simulink model "SCADA"  (R2025a)
settings: Solver=FixedStepAuto  StartTime=0.0  StopTime=inf  FixedStep=0.001  RelTol=1e-3
InitFcn:
  | addpath('SCADA');
  | initFcn_SCADA;
model workspace (MAT data in the model file):
  RadSysCoeff = Simulink.Parameter
  RadSysCoeff.Value = [1 2 3 4]
  RadSysCoeff.Complexity = 'real'
  RadSysCoeff.Dimensions = [1 4]
  RadSysCoeff.DataType = 'auto'
undefined symbols (not defined in the file): daq, g, HIL_act_A_cap, HIL_act_A_rod, HIL_charge_ki, HIL_charge_kp, HIL_charge_nMax, HIL_charge_nMin, HIL_ERU_kd, HIL_ERU_ki, HIL_ERU_kp, HIL_ERU_nMax, HIL_gen_kd, HIL_gen_ki, HIL_gen_kp, HIL_gen_nMax, HIL_gen_nMin, HIL_H1T_kd, HIL_H1T_ki, HIL_H1T_kp, HIL_H1T_P1fBias, HIL_H1T_P1negCutIn, HIL_H1T_P1posCutIn, HIL_H1T_P2fBias, HIL_H1T_P2negCutIn, HIL_H1T_P2posCutIn, HIL_scale_sys, HIL_WECpump_A_cap, HIL_WECpump_A_rod, HIL_WECpump_ang2lin, HIL_WECpump_negativeCtrlLimit, HIL_WECpump_positiveCtrlLimit, National_Instruments, PCIe, rho, wave_phi, wave_S_w, WEC_A_rad, WEC_B_rad, WEC_dw, WEC_F_amp, WEC_h, WEC_I, WEC_I_inf, WEC_ICs, WEC_L_cm, WEC_L_flap, WEC_m, WEC_phi_e, WEC_T, WEC_W, WEC_w
libraries: sldrtlib x26, slpidlib x4, daqlib x1, simulink x1
(part 1 of 2)
settings Model: Creator=Jeremy  LastModifiedBy=wills224
settings DataIOCC: SaveFormat=Structure  ReturnWorkspaceOutputs=off  TimeSaveName=time  SignalLoggingName=out
settings DebuggingCC: UnderspecifiedInitializationDetection=Classic  MergeDetectMultiDrivingBlocksExec=none  UnconnectedInputMsg=warning  UnconnectedOutputMsg=warning  UnconnectedLineMsg=warning
settings ModelReferenceCC: EnableRefExpFcnMdlSchedulingChecks=on  PropagateSignalLabelsOutOfModel=off
settings RTWCC: GPUComputeCapability=3.5  DLArmComputeVersion=19.05

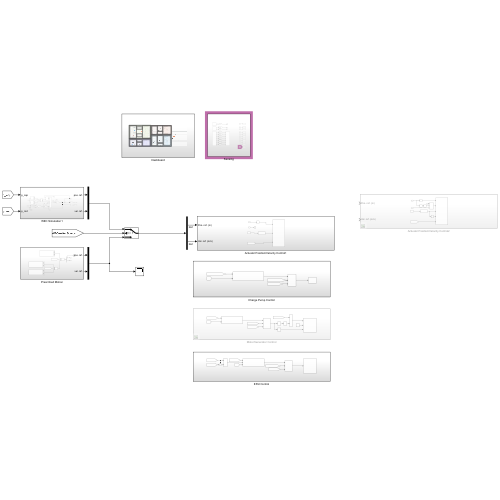
[thumbnail: Simulink's stored preview of the top-level diagram]
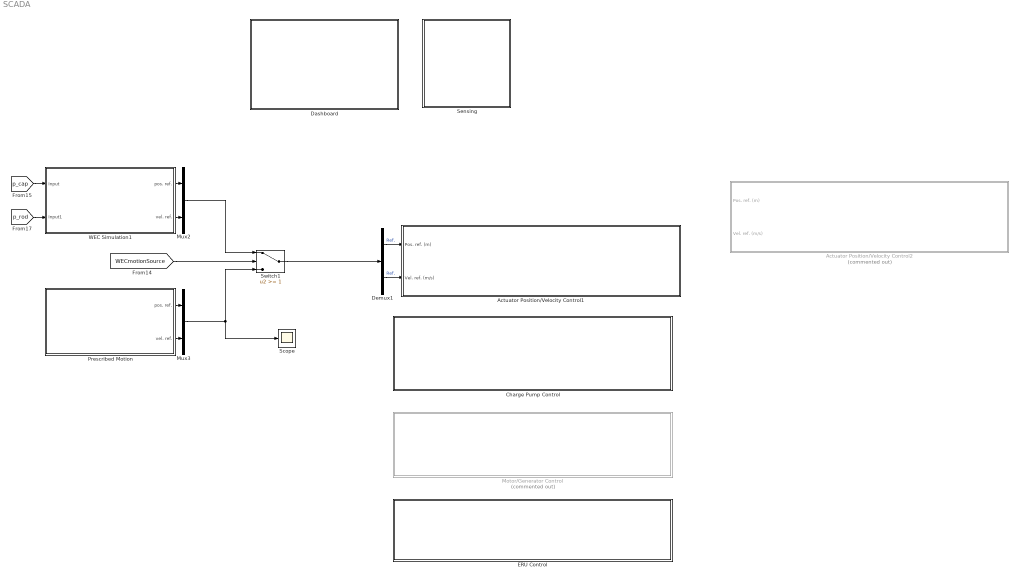
== system SCADA ==
  Actuator Position/Velocity Control1 : Subsystem
  Actuator Position/Velocity Control2 : Subsystem  Commented=on
  Charge Pump Control : Subsystem
  Dashboard : Subsystem
  Demux1 : Demux  Outputs=2
  ERU Control : Subsystem
  Motor/Generator Control : Subsystem  Commented=on
  Mux2 : Mux  Inputs=2
  Mux3 : Mux  Inputs=2
  Prescribed Motion : Subsystem
  Scope : Scope
      settings: ActiveDisplayYMinimum=-0.0625  ActiveDisplayYMaximum=0.0625  DataLoggingVariableName=ScopeData12
  Sensing : Subsystem
  Switch1 : Switch  Threshold=1  SaturateOnIntegerOverflow=off  InputSameDT=off
  WEC Simulation1 : Subsystem
  wires:
  WEC Simulation1/2(vel. ref.) -> Mux2/2
  [p_cap] -> WEC Simulation1/1(Input)
  Prescribed Motion/2(vel. ref.) -> Mux3/2
  Switch1/1 -> Demux1/1
  Demux1/2 -> Actuator Position/Velocity Control1/2(Vel. ref. (m/s))  "Ref."
  Prescribed Motion/1(pos. ref.) -> Mux3/1
  Mux3/1 -> Scope/1, Switch1/3
  [p_rod] -> WEC Simulation1/2(Input1)
  [WECmotionSource] -> Switch1/2
  WEC Simulation1/1(pos. ref.) -> Mux2/1
  Mux2/1 -> Switch1/1
  Demux1/1 -> Actuator Position/Velocity Control1/1(Pos. ref. (m))  "Ref."

== system SCADA/Actuator Position//Velocity Control1 ==
  Pos. ref. (m) : Inport
  Vel. ref. (m/s) : Inport  Port=2
  Saturation : Saturate  UpperLimit=HIL_WECpump_positiveCtrlLimit  LowerLimit=HIL_WECpump_negativeCtrlLimit
  Subsystem : Subsystem
  Terminator : Terminator
  Transfer Fcn1 : TransferFcn  Denominator=[0.001 1]
  wires:
  [x_wp] -> Transfer Fcn1/1
  Pos. ref. (m)/1 -> Saturation/1
  [H1T_shaftSpeed] -> Subsystem/3(H1T shaft speed (rpm))
  Transfer Fcn1/1 -> Subsystem/2(Pos. meas. (m))
  Saturation/1 -> Subsystem/1(Pos. ref. (m))
  Vel. ref. (m/s)/1 -> Terminator/1

== system SCADA/Actuator Position//Velocity Control2 ==
  Pos. ref. (m) : Inport
  Vel. ref. (m/s) : Inport  Port=2
  Abs : Abs  SaturateOnIntegerOverflow=off
  Constant : Constant  Value=0
  Dead Zone : DeadZone  LowerValue=HIL_WECpump_negativeCtrlLimit  UpperValue=HIL_WECpump_positiveCtrlLimit
  Derivative : Derivative
  Saturation : Saturate  UpperLimit=HIL_WECpump_positiveCtrlLimit  LowerLimit=HIL_WECpump_negativeCtrlLimit
  Subsystem : Subsystem
  Switch1 : Switch  Criteria=u2 > Threshold  SaturateOnIntegerOverflow=off  InputSameDT=off
  Transfer Fcn1 : TransferFcn  Denominator=[0.001 1]
  wires:
  Vel. ref. (m/s)/1 -> Switch1/3
  Switch1/1 -> Subsystem/2(Vel. ref. (m/s))
  Constant/1 -> Switch1/1
  Abs/1 -> Switch1/2
  Dead Zone/1 -> Abs/1
  Saturation/1 -> Subsystem/1(Pos. ref. (m))
  Transfer Fcn1/1 -> Derivative/1, Subsystem/3(Pos. meas. (m))
  [H1T_shaftSpeed] -> Subsystem/5(H1T shaft speed (rpm))
  Derivative/1 -> Subsystem/4(Vel. meas. (m/s))
  Pos. ref. (m)/1 -> Dead Zone/1, Saturation/1
  [x_wp] -> Transfer Fcn1/1

== system SCADA/Charge Pump Control ==
  Low-pressure manifold pressure control : Subsystem
  Switch : Switch  Criteria=u2 > Threshold  SaturateOnIntegerOverflow=off  InputSameDT=off
  charge pump : Subsystem
  wires:
  [p_l] -> Low-pressure manifold pressure control/2(pressure meas. (Pa))
  [ChargePumpSpeed] -> Switch/3
  [LPManifoldPressureRef] -> Low-pressure manifold pressure control/1(pressure ref. (Pa))
  Low-pressure manifold pressure control/1(charge pump shaft speed (rpm)) -> Switch/1
  [ChargePumpSpeedOrPressure] -> Switch/2
  Switch/1 -> charge pump/1(Speed ref.)

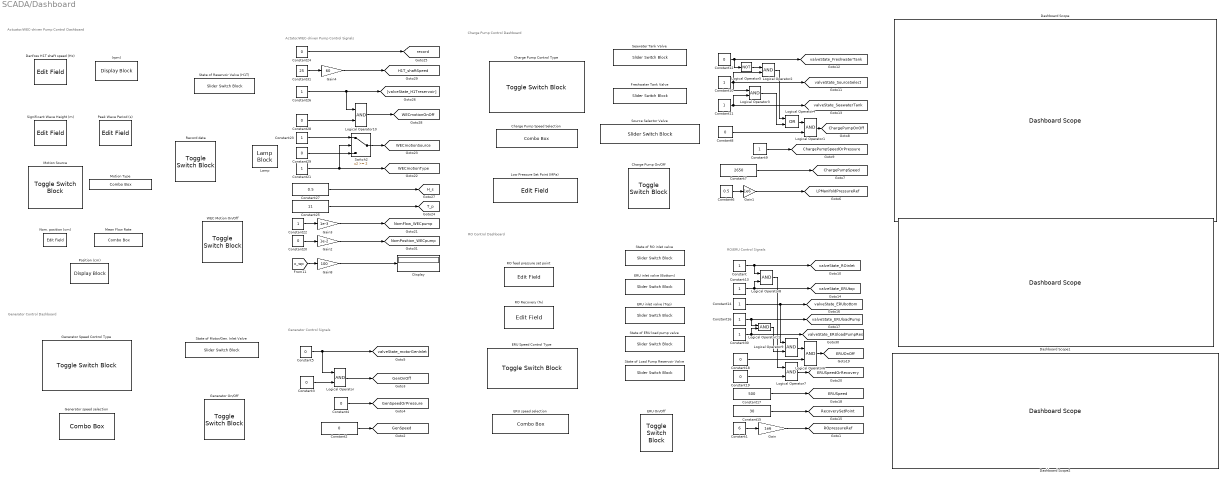
== system SCADA/Dashboard ==
  note: Charge Pump Control Dashboard
  note: Generator Control Signals
  note: RO Control Dashboard
  note: Generator Control Dashboard
  note: RO/ERU Control Signals
  note: Actator/WEC-driven Pump Control Signals
  note: Actuator/WEC-driven Pump Control Dashboard
  (rpm) : DisplayBlock  LabelPosition=Hide  Format=long  Transparency=1  GridColor=[0.502, 0.502, 0.502]
  Charge Pump Control Type : ToggleSwitchBlock  LabelPosition=Hide
  Charge Pump On/Off : ToggleSwitchBlock  LabelPosition=Hide
  Charge Pump Speed Selection : ComboBox  LabelPosition=Hide  SelectedLabel=2650 rpm
  Constant{,9..11,13..14,16,21..23,26,30} (12 alike) : Constant
  Constant1 : Constant  Value=6
  Constant{2..5,8,12,18..20,24,28..29} (12 alike) : Constant  Value=0
  Constant15 : Constant  Value=30
  Constant17 : Constant  Value=500
  Constant25 : Constant  Value=11
  Constant27 : Constant  Value=0.5
  Constant31 : Constant  Value=25
  Constant6 : Constant  Value=0.5
  Constant7 : Constant  Value=2650
  Danfoss H1T shaft speed (Hz) : EditField  LabelPosition=Hide  ShowInitialText=on  Alignment=Center
  Dashboard Scope : DashboardScope  ShowInitialText=off  FontColor=[0.0, 0.0, 0.0]
  Dashboard Scope1 : DashboardScope  FontColor=[0.0, 0.0, 0.0]
  Dashboard Scope2 : DashboardScope  FontColor=[0.0, 0.0, 0.0]
  Display : Display
  ERU On/Off : ToggleSwitchBlock  LabelPosition=Hide
  ERU Speed Control Type : ToggleSwitchBlock  LabelPosition=Hide
  ERU inlet valve (Bottom) : SliderSwitchBlock  LabelPosition=Hide
  ERU inlet valve (Top) : SliderSwitchBlock  LabelPosition=Hide
  ERU speed selection : ComboBox  LabelPosition=Hide  SelectedLabel=500 rpm
  Freshwater Tank Valve : SliderSwitchBlock  LabelPosition=Hide
  Gain : Gain  Gain=1e6
  Gain1 : Gain  Gain=1e6
  Gain2 : Gain  Gain=1e-2
  Gain3 : Gain  Gain=1e-3
  Gain4 : Gain  Gain=60
  Gain8 : Gain  Gain=100
  Generator On/Off : ToggleSwitchBlock  LabelPosition=Hide
  Generator Speed Control Type : ToggleSwitchBlock  LabelPosition=Hide
  Generator speed selection : ComboBox  LabelPosition=Hide  SelectedLabel=0 rpm
  Lamp : LampBlock  LabelPosition=Hide  DefaultColor=[192.0, 192.0, 192.0]
  Logical Operator{,1..3,6..11} (10 alike) : Logic  AllPortsSameDT=off  OutDataTypeStr=boolean
  Logical Operator4 : Logic  Operator=OR  AllPortsSameDT=off  OutDataTypeStr=boolean
  Logical Operator5 : Logic  Operator=NOT  AllPortsSameDT=off  OutDataTypeStr=boolean
  Low Pressure Set Point (MPa) : EditField  LabelPosition=Hide  ShowInitialText=on  Alignment=Center
  Mean Flow Rate : ComboBox  LabelPosition=Hide  SelectedLabel=1 L/s
  Motion Source : ToggleSwitchBlock  LabelPosition=Hide
  Motion Type : ComboBox  LabelPosition=Hide  SelectedLabel=Position, Constant
  Nom. position (cm) : EditField  LabelPosition=Hide  ShowInitialText=on  Alignment=Center
  Peak Wave Period (s) : EditField  LabelPosition=Hide  ShowInitialText=on  Alignment=Center
  Position (cm) : DisplayBlock  LabelPosition=Hide  Format=long  Transparency=1  GridColor=[0.502, 0.502, 0.502]
  RO Recovery (%) : EditField  LabelPosition=Hide  ShowInitialText=on  Alignment=Center
  RO feed pressure set point : EditField  LabelPosition=Hide  ShowInitialText=on  Alignment=Center
  Record data : ToggleSwitchBlock  LabelPosition=Hide
  Seawater Tank Valve : SliderSwitchBlock  LabelPosition=Hide
  Significant Wave Height (m) : EditField  LabelPosition=Hide  ShowInitialText=on  Alignment=Center
  Source Selector Valve : SliderSwitchBlock  LabelPosition=Hide
  State of ERU load pump valve : SliderSwitchBlock  LabelPosition=Hide
  State of Load Pump Reservoir Valve : SliderSwitchBlock  LabelPosition=Hide
  State of Motor/Gen. Inlet Valve : SliderSwitchBlock  LabelPosition=Hide
  State of RO inlet valve : SliderSwitchBlock  LabelPosition=Hide
  State of Reservoir Valve (H1T) : SliderSwitchBlock  LabelPosition=Hide
  Switch2 : Switch  Threshold=2  SaturateOnIntegerOverflow=off  InputSameDT=off
  WEC Motion On/Off : ToggleSwitchBlock  LabelPosition=Hide
  tag scope: ChargePumpOnOff=global, ChargePumpSpeed=global, ChargePumpSpeedOrPressure=global, ERUOnOff=global, ERUSpeed=global, ERUSpeedOrRecovery=global, GenOnOff=global, GenSpeed=global, GenSpeedOrPressure=global, H1T_shaftSpeed=global, H_s=global, LPManifoldPressureRef=global, NomFlow_WECpump=global, NomPosition_WECpump=global, ROpressureRef=global, RecoverySetPoint=global, T_p=global, WECmotionOnOff=global, WECmotionSource=global, WECmotionType=global, record=global, valveState_ERUbottom=global, valveState_ERUloadPump=global, valveState_ERUloadPumpRes=global, valveState_ERUtop=global, valveState_FreshwaterTank=global, valveState_ROinlet=global, valveState_SeawaterTank=global, valveState_SourceSelect=global, valveState_motorGenInlet=global
  wires:
  Constant/1 -> Logical Operator8/1, [valveState_ROinlet]
  Constant1/1 -> Gain/1
  Constant2/1 -> [GenSpeed]
  Constant3/1 -> Logical Operator/2
  Constant4/1 -> [GenSpeedOrPressure]
  Constant5/1 -> Logical Operator/1, [valveState_motorGenInlet]
  Logical Operator/1 -> [GenOnOff]
  Logical Operator1/1 -> [ChargePumpOnOff]
  Constant9/1 -> [ChargePumpSpeedOrPressure]
  Constant10/1 -> [valveState_SourceSelect], Logical Operator2/2, Logical Operator3/1
  Gain1/1 -> [LPManifoldPressureRef]
  Constant6/1 -> Gain1/1
  Constant8/1 -> Logical Operator1/2
  Constant7/1 -> [ChargePumpSpeed]
  Constant12/1 -> Logical Operator5/1, [valveState_FreshwaterTank]
  Constant11/1 -> Logical Operator3/2, [valveState_SeawaterTank]
  Logical Operator4/1 -> Logical Operator1/1
  Logical Operator3/1 -> Logical Operator4/2
  Logical Operator2/1 -> Logical Operator4/1
  Logical Operator5/1 -> Logical Operator2/1
  Logical Operator6/1 -> [ERUOnOff]
  Constant17/1 -> [ERUSpeed]
  Constant13/1 -> Logical Operator8/2, [valveState_ERUtop]
  Constant19/1 -> Logical Operator7/2
  Constant18/1 -> Logical Operator6/2
  Constant14/1 -> [valveState_ERUbottom], Logical Operator9/1
  Constant15/1 -> [RecoverySetPoint]
  Logical Operator7/1 -> [ERUSpeedOrRecovery]
  Logical Operator8/1 -> Logical Operator7/1
  Logical Operator9/1 -> Logical Operator6/1
  Constant16/1 -> [valveState_ERUloadPump], Logical Operator11/1
  Constant30/1 -> [valveState_ERUloadPumpRes], Logical Operator11/2
  Logical Operator11/1 -> Logical Operator9/2
  Gain4/1 -> [H1T_shaftSpeed]
  Constant28/1 -> Logical Operator10/2
  Constant31/1 -> Gain4/1
  Gain3/1 -> [NomFlow_WECpump]
  Logical Operator10/1 -> [WECmotionOnOff]
  Switch2/1 -> [WECmotionSource]
  Constant27/1 -> [H_s]
  Constant24/1 -> [record]
  Constant26/1 -> Logical Operator10/1, [valveState_H1Treservoir]
  Constant22/1 -> Gain3/1
  Gain2/1 -> [NomPosition_WECpump]
  Constant23/1 -> Switch2/1
  Constant29/1 -> Switch2/3
  Constant21/1 -> Switch2/2, [WECmotionType]
  Constant20/1 -> Gain2/1
  Constant25/1 -> [T_p]
  Gain8/1 -> Display/1
  [x_wp] -> Gain8/1
  Gain/1 -> [ROpressureRef]

== system SCADA/ERU Control ==
  Divide : Product  Inputs=*/
  ERU : Subsystem
  RO control : Subsystem
  Sum : Sum  Inputs=++|
  Switch : Switch  Criteria=u2 > Threshold  SaturateOnIntegerOverflow=off  InputSameDT=off
  wires:
  [p_f] -> RO control/3(feed pressure (Pa))
  [q_perm] -> Sum/1, Divide/1
  [q_brine] -> Sum/2
  Sum/1 -> Divide/2
  [RecoverySetPoint] -> RO control/1(recovery ref.)
  Divide/1 -> RO control/2(recovery meas.)
  [ERUSpeedOrRecovery] -> Switch/2
  [ERUSpeed] -> Switch/3
  RO control/1(ERU shaft speed (rpm)) -> Switch/1
  Switch/1 -> ERU/1(Speed ref.)

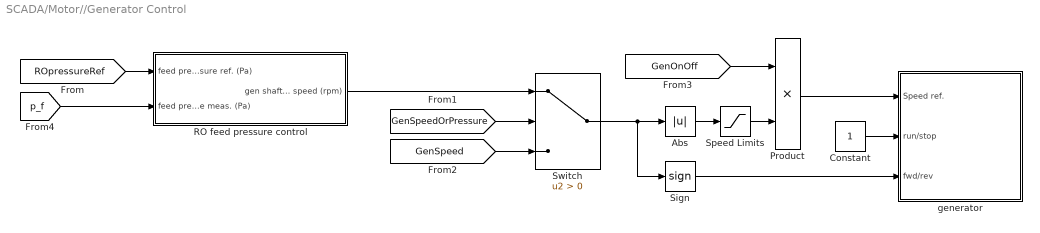
== system SCADA/Motor//Generator Control ==
  Abs : Abs  SaturateOnIntegerOverflow=off
  Constant : Constant
  Product : Product
  RO feed pressure control : Subsystem
  Sign : Signum
  Speed Limits : Saturate  UpperLimit=HIL_gen_nMax  LowerLimit=HIL_gen_nMin
  Switch : Switch  Criteria=u2 > Threshold  SaturateOnIntegerOverflow=off  InputSameDT=off
  generator : Subsystem
  wires:
  RO feed pressure control/1(gen shaft speed (rpm)) -> Switch/1
  [p_f] -> RO feed pressure control/2(feed pressure meas. (Pa))
  [ROpressureRef] -> RO feed pressure control/1(feed pressure ref. (Pa))
  Switch/1 -> Sign/1, Abs/1
  [GenSpeedOrPressure] -> Switch/2
  [GenSpeed] -> Switch/3
  [GenOnOff] -> Product/1
  Product/1 -> generator/1(Speed ref.)
  Constant/1 -> generator/2(run/stop)
  Sign/1 -> generator/3(fwd/rev)
  Speed Limits/1 -> Product/2
  Abs/1 -> Speed Limits/1

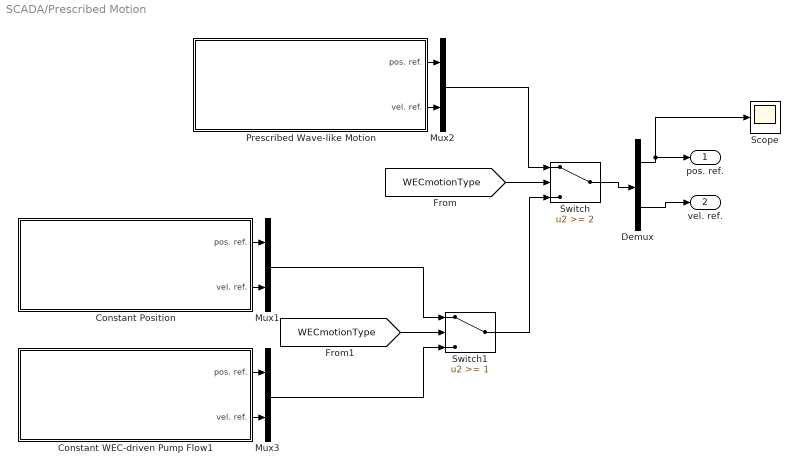
== system SCADA/Prescribed Motion ==
  Constant Position : Subsystem
  Constant WEC-driven Pump Flow1 : Subsystem
  Demux : Demux  Outputs=2
  Mux1 : Mux  Inputs=2
  Mux2 : Mux  Inputs=2
  Mux3 : Mux  Inputs=2
  Prescribed Wave-like Motion : Subsystem
  Scope : Scope
      settings: ActiveDisplayYMinimum=-0.0012499999999999976  ActiveDisplayYMaximum=0.11125  DataLoggingVariableName=ScopeData13
  Switch : Switch  Threshold=2  SaturateOnIntegerOverflow=off  InputSameDT=off
  Switch1 : Switch  Threshold=1  SaturateOnIntegerOverflow=off  InputSameDT=off
  pos. ref. : Outport
  vel. ref. : Outport  Port=2
  wires:
  Prescribed Wave-like Motion/2(vel. ref.) -> Mux2/2
  Prescribed Wave-like Motion/1(pos. ref.) -> Mux2/1
  Mux2/1 -> Switch/1
  Demux/2 -> vel. ref./1
  Demux/1 -> Scope/1, pos. ref./1
  Constant Position/1(pos. ref.) -> Mux1/1
  Constant Position/2(vel. ref.) -> Mux1/2
  [WECmotionType] -> Switch/2
  Switch/1 -> Demux/1
  Constant WEC-driven Pump Flow1/2(vel. ref.) -> Mux3/2
  Constant WEC-driven Pump Flow1/1(pos. ref.) -> Mux3/1
  Mux3/1 -> Switch1/3
  [WECmotionType] -> Switch1/2
  Switch1/1 -> Switch/3
  Mux1/1 -> Switch1/1

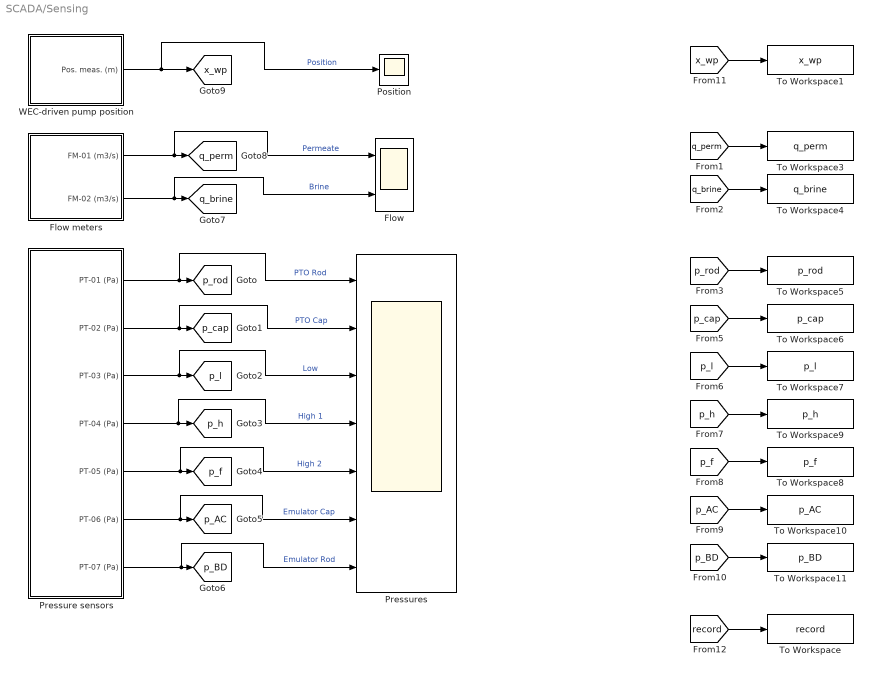
== system SCADA/Sensing ==
  Flow : Scope  NumInputPorts=2
      settings: DataLoggingVariableName=ScopeData14
  Flow meters : Subsystem
  Position : Scope
      settings: ActiveDisplayYMinimum=0.0011982402807289294  ActiveDisplayYMaximum=0.0033569285576201258  DataLoggingVariableName=ScopeData22
  Pressure sensors : Subsystem
  Pressures : Scope  NumInputPorts=7
      settings: ActiveDisplayYMinimum=-1.1076278561771905E+7  ActiveDisplayYMaximum=795336.49775385088
  To Workspace : ToWorkspace  VariableName=record  SaveFormat=Timeseries  SampleTime=-1
  To Workspace1 : ToWorkspace  VariableName=x_wp  SaveFormat=Timeseries  SampleTime=-1
  To Workspace10 : ToWorkspace  VariableName=p_AC  SaveFormat=Timeseries  SampleTime=-1
  To Workspace11 : ToWorkspace  VariableName=p_BD  SaveFormat=Timeseries  SampleTime=-1
  To Workspace3 : ToWorkspace  VariableName=q_perm  SaveFormat=Timeseries  SampleTime=-1
  To Workspace4 : ToWorkspace  VariableName=q_brine  SaveFormat=Timeseries  SampleTime=-1
  To Workspace5 : ToWorkspace  VariableName=p_rod  SaveFormat=Timeseries  SampleTime=-1
  To Workspace6 : ToWorkspace  VariableName=p_cap  SaveFormat=Timeseries  SampleTime=-1
  To Workspace7 : ToWorkspace  VariableName=p_l  SaveFormat=Timeseries  SampleTime=-1
  To Workspace8 : ToWorkspace  VariableName=p_f  SaveFormat=Timeseries  SampleTime=-1
  To Workspace9 : ToWorkspace  VariableName=p_h  SaveFormat=Timeseries  SampleTime=-1
  WEC-driven pump position : Subsystem
  tag scope: p_AC=global, p_BD=global, p_cap=global, p_f=global, p_h=global, p_l=global, p_rod=global, q_brine=global, q_perm=global, x_wp=global
  wires:
  [p_l] -> To Workspace7/1
  [p_cap] -> To Workspace6/1
  [p_h] -> To Workspace9/1
  [q_perm] -> To Workspace3/1
  [p_AC] -> To Workspace10/1
  [p_BD] -> To Workspace11/1
  [p_f] -> To Workspace8/1
  Pressure sensors/1(PT-01 (Pa)) -> Pressures/1, [p_rod]  "PTO Rod"
  Pressure sensors/4(PT-04 (Pa)) -> Pressures/4, [p_h]  "High 1"
  [q_brine] -> To Workspace4/1
  [p_rod] -> To Workspace5/1
  [x_wp] -> To Workspace1/1
  Pressure sensors/2(PT-02 (Pa)) -> Pressures/2, [p_cap]  "PTO Cap"
  [record] -> To Workspace/1
  Flow meters/2(FM-02 (m3/s)) -> Flow/2, [q_brine]  "Brine"
  Pressure sensors/3(PT-03 (Pa)) -> [p_l], Pressures/3  "Low"
  Pressure sensors/6(PT-06 (Pa)) -> Pressures/6, [p_AC]  "Emulator Cap"
  Pressure sensors/7(PT-07 (Pa)) -> Pressures/7, [p_BD]  "Emulator Rod"
  WEC-driven pump position/1(Pos. meas. (m)) -> Position/1, [x_wp]  "Position"
  Flow meters/1(FM-01 (m3/s)) -> Flow/1, [q_perm]  "Permeate"
  Pressure sensors/5(PT-05 (Pa)) -> Pressures/5, [p_f]  "High 2"

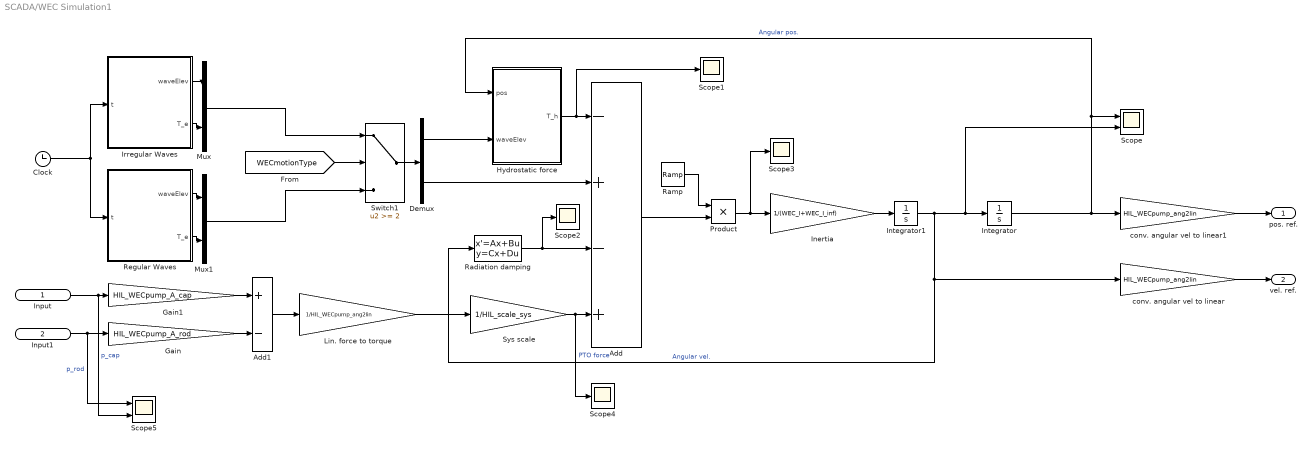
== system SCADA/WEC Simulation1 ==
  Input : Inport  SampleTime=0.01
  Input1 : Inport  Port=2  SampleTime=0.01
  Add : Sum  Inputs=-+-+
  Add1 : Sum  Inputs=+-
  Clock : Clock
  Demux : Demux  Outputs=2
  Gain : Gain  Gain=HIL_WECpump_A_rod
  Gain1 : Gain  Gain=HIL_WECpump_A_cap
  Hydrostatic force : MATLAB Function  TreatAsAtomicUnit=on
  Inertia : Gain  Gain=1/(WEC_I+WEC_I_inf)
  Integrator : Integrator
  Integrator1 : Integrator
  Irregular Waves : MATLAB Function  TreatAsAtomicUnit=on
  Lin. force to torque : Gain  Gain=1/HIL_WECpump_ang2lin
  Mux : Mux  Inputs=2
  Mux1 : Mux  Inputs=2
  Product : Product
  Radiation damping : StateSpace  A=WEC_A_rad  B=WEC_B_rad  C=[1,0,0]  D=0  InitialCondition=WEC_ICs
  Ramp : simulink/Sources/Ramp  slope=1/5  start=0.5  InitialOutput=0
  Regular Waves : MATLAB Function  TreatAsAtomicUnit=on
  Scope : Scope  NumInputPorts=2
      settings: DataLoggingSaveFormat=Array
  Scope{1..4} (4 alike) : Scope
      Scope1 settings: DataLoggingVariableName=ScopeData2  DataLoggingSaveFormat=Array
      Scope2 settings: DataLoggingVariableName=ScopeData3  DataLoggingSaveFormat=Array
      Scope3 settings: DataLoggingVariableName=ScopeData4  DataLoggingSaveFormat=Array
      Scope4 settings: DataLoggingVariableName=ScopeData5  DataLoggingSaveFormat=Array
  Scope5 : Scope  NumInputPorts=2
      settings: DataLoggingVariableName=ScopeData6  DataLoggingSaveFormat=Array
  Switch1 : Switch  Threshold=2  SaturateOnIntegerOverflow=off  InputSameDT=off
  Sys scale : Gain  Gain=1/HIL_scale_sys
  conv. angular vel to linear : Gain  Gain=HIL_WECpump_ang2lin
  conv. angular vel to linear1 : Gain  Gain=HIL_WECpump_ang2lin
  pos. ref. : Outport
  vel. ref. : Outport  Port=2
  wires:
  Radiation damping/1 -> Add/3, Scope2/1
  Clock/1 -> Regular Waves/1(t), Irregular Waves/1(t)
  Irregular Waves/1(waveElev) -> Mux/1
  Irregular Waves/2(T_e) -> Mux/2
  Hydrostatic force/1(T_h) -> Scope1/1, Add/1
  Inertia/1 -> Integrator1/1
  Integrator1/1 -> Scope/2, Integrator/1, Radiation damping/1, conv. angular vel to linear/1  "Angular vel."
  Integrator/1 -> conv. angular vel to linear1/1, Scope/1, Hydrostatic force/1(pos)  "Angular pos."
  Lin. force to torque/1 -> Sys scale/1
  Add1/1 -> Lin. force to torque/1
  Input/1 -> Scope5/2, Gain1/1  "p_cap"
  Input1/1 -> Scope5/1, Gain/1  "p_rod"
  conv. angular vel to linear1/1 -> pos. ref./1
  conv. angular vel to linear/1 -> vel. ref./1
  Sys scale/1 -> Add/4, Scope4/1  "PTO force"
  Gain/1 -> Add1/2
  Gain1/1 -> Add1/1
  Demux/1 -> Hydrostatic force/2(waveElev)
  [WECmotionType] -> Switch1/2
  Demux/2 -> Add/2
  Regular Waves/1(waveElev) -> Mux1/1
  Regular Waves/2(T_e) -> Mux1/2
  Switch1/1 -> Demux/1
  Mux1/1 -> Switch1/3
  Mux/1 -> Switch1/1
  Product/1 -> Scope3/1, Inertia/1
  Add/1 -> Product/2
  Ramp/1 -> Product/1

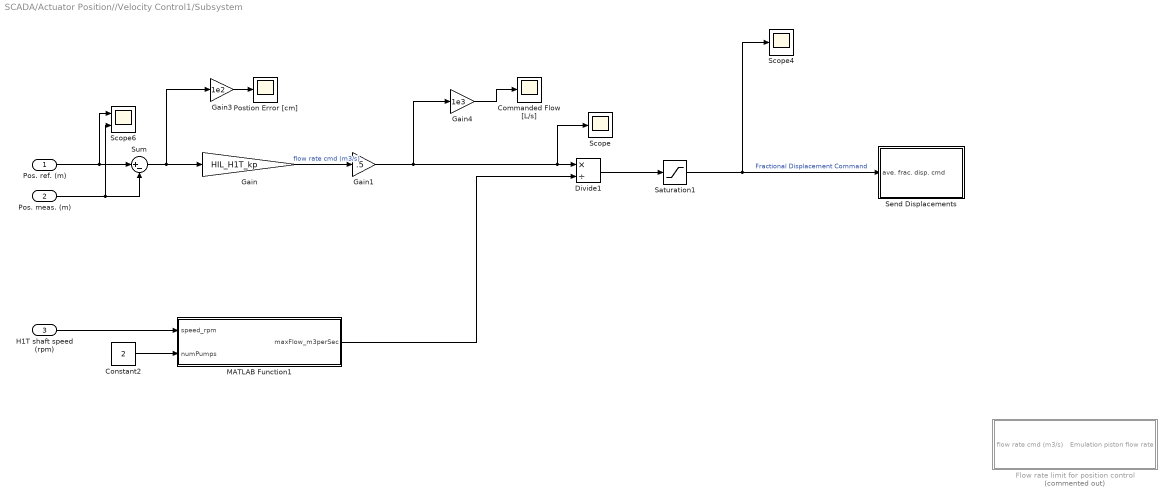
== system SCADA/Actuator Position//Velocity Control1/Subsystem ==
  Pos. ref. (m) : Inport  SampleTime=0.01
  Pos. meas. (m) : Inport  Port=2  SampleTime=0.01
  H1T shaft speed (rpm) : Inport  Port=3
  Commanded Flow [L/s] : Scope
      settings: ActiveDisplayYMinimum=-7.5975236079021844  ActiveDisplayYMaximum=7.6371479012594943  DataLoggingVariableName=ScopeData17
  Constant2 : Constant  Value=2
  Divide1 : Product  Inputs=*/
  Flow rate limit for position control : Subsystem  Commented=on
  Gain : Gain  Gain=HIL_H1T_kp
  Gain1 : Gain  Gain=.5
  Gain3 : Gain  Gain=1e2
  Gain4 : Gain  Gain=1e3
  MATLAB Function1 : MATLAB Function  TreatAsAtomicUnit=on
  Postion Error [cm] : Scope
      settings: ActiveDisplayYMinimum=-12.877251579571915  ActiveDisplayYMaximum=12.868133706587805  DataLoggingVariableName=ScopeData15
  Saturation1 : Saturate  UpperLimit=1  LowerLimit=-1
  Scope : Scope
      settings: ActiveDisplayYMinimum=-0.00010203992147228588  ActiveDisplayYMaximum=-3.1811275053556521E-5  DataLoggingVariableName=ScopeData25
  Scope4 : Scope
      settings: ActiveDisplayYMinimum=-1.25  ActiveDisplayYMaximum=1.25  DataLoggingVariableName=ScopeData16
  Scope6 : Scope  NumInputPorts=2
      settings: ActiveDisplayYMinimum=-0.077105111095338921  ActiveDisplayYMaximum=0.068463787942577917  DataLoggingVariableName=ScopeData21
  Send Displacements : Subsystem
  Sum : Sum  Inputs=|+-
  wires:
  Pos. meas. (m)/1 -> Scope6/2, Sum/2
  MATLAB Function1/1(maxFlow_m3perSec) -> Divide1/2
  Constant2/1 -> MATLAB Function1/2(numPumps)
  Divide1/1 -> Saturation1/1
  H1T shaft speed (rpm)/1 -> MATLAB Function1/1(speed_rpm)
  Pos. ref. (m)/1 -> Scope6/1, Sum/1
  Sum/1 -> Gain/1, Gain3/1
  Gain/1 -> Gain1/1  "flow rate cmd (m3/s)"
  Gain3/1 -> Postion Error [cm]/1
  Gain4/1 -> Commanded Flow [L/s]/1
  Gain1/1 -> Scope/1, Divide1/1, Gain4/1
  Saturation1/1 -> Send Displacements/1(ave. frac. disp. cmd), Scope4/1  "Fractional Displacement Command"

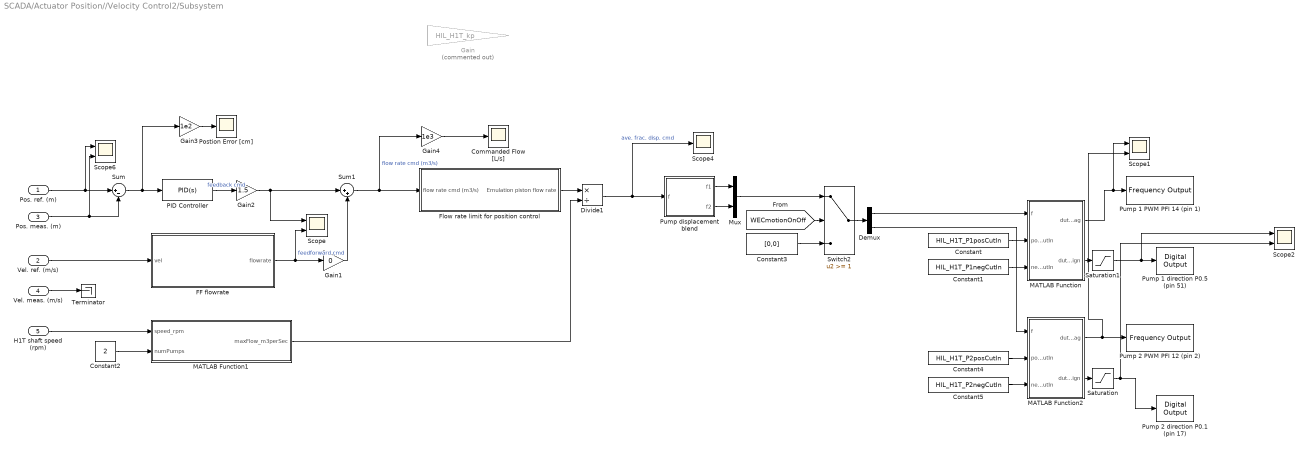
== system SCADA/Actuator Position//Velocity Control2/Subsystem ==
  Pos. ref. (m) : Inport  SampleTime=0.01
  Vel. ref. (m/s) : Inport  Port=2  SampleTime=0.01
  Pos. meas. (m) : Inport  Port=3  SampleTime=0.01
  Vel. meas. (m/s) : Inport  Port=4  SampleTime=0.01
  H1T shaft speed (rpm) : Inport  Port=5
  Commanded Flow [L/s] : Scope
      settings: ActiveDisplayYMinimum=-5.6250000000000009  ActiveDisplayYMaximum=5.6250000000000009  DataLoggingVariableName=ScopeData17
  Constant : Constant  Value=HIL_H1T_P1posCutIn
  Constant1 : Constant  Value=HIL_H1T_P1negCutIn
  Constant2 : Constant  Value=2
  Constant3 : Constant  Value=[0,0]
  Constant4 : Constant  Value=HIL_H1T_P2posCutIn
  Constant5 : Constant  Value=HIL_H1T_P2negCutIn
  Demux : Demux  Outputs=2
  Divide1 : Product  Inputs=*/
  FF flowrate : MATLAB Function  TreatAsAtomicUnit=on
  Flow rate limit for position control : Subsystem
  Gain : Gain  Commented=on  Gain=HIL_H1T_kp
  Gain1 : Gain  Gain=0
  Gain2 : Gain  Gain=1.5
  Gain3 : Gain  Gain=1e2
  Gain4 : Gain  Gain=1e3
  MATLAB Function : MATLAB Function  TreatAsAtomicUnit=on
  MATLAB Function1 : MATLAB Function  TreatAsAtomicUnit=on
  MATLAB Function2 : MATLAB Function  TreatAsAtomicUnit=on
  Mux : Mux  Inputs=2
  PID Controller : slpidlib/PID Controller  Controller=PID  Form=Parallel  TimeDomain=Continuous-time  UseExternalTs=off  SampleTime=-1  IntegratorMethod=Forward Euler  FilterMethod=Forward Euler  ControllerParametersSource=internal  P=HIL_H1T_kp  I=HIL_H1T_ki  UseKiTs=off  D=HIL_H1T_kd  UseExternalDerivativeSource=off  N=100  UseFilter=on  TunerSelectOption=Transfer Function Based (PID Tuner App)  InitialConditionSource=internal  InitialConditionForIntegrator=0  InitialConditionForFilter=0  DifferentiatorICPrevScaledInput=0  ExternalReset=none  TrackingMode=off  Kt=50  LimitOutput=on  SatLimitsSource=internal  UpperSaturationLimit=0.003  LowerSaturationLimit=-0.003  LinearizeAsGain=on  AntiWindupMode=none  Kb=10  LimitIntegrator=on  UpperIntegratorSaturationLimit=.01  LowerIntegratorSaturationLimit=-.01  POutMin=[]  POutMax=[]  IOutMin=[]  IOutMax=[]  DOutMin=[]  DOutMax=[]  NOutMin=[]  NOutMax=[]  SumOutMin=[]  SumOutMax=[]  SaturationOutMin=[]  SaturationOutMax=[]  PParamMin=[]  PParamMax=[]  IParamMin=[]  IParamMax=[]  DParamMin=[]  DParamMax=[]  NParamMin=[]  NParamMax=[]  KbParamMin=[]  KbParamMax=[]  KtParamMin=[]  KtParamMax=[]  KbOutMin=[]  KbOutMax=[]  KtOutMin=[]  KtOutMax=[]  IntegratorOutMin=[]  IntegratorOutMax=[]  FilterOutMin=[]  FilterOutMax=[]  SumI1OutMin=[]  SumI1OutMax=[]  SumI2OutMin=[]  SumI2OutMax=[]  SumI3OutMin=[]  SumI3OutMax=[]  SumI4OutMin=[]  SumI4OutMax=[]  SumDOutMin=[]  SumDOutMax=[]  DifferentiatorOutMin=[]  DifferentiatorOutMax=[]  FilterDiffOutCoefMin=[]  FilterDiffOutCoefMax=[]  ReciprocalOutMin=[]  ReciprocalOutMax=[]  SumDenOutMin=[]  SumDenOutMax=[]  SumNumOutMin=[]  SumNumOutMax=[]  DivideOutMin=[]  DivideOutMax=[]  UdiffTsProdOutMin=[]  UdiffTsProdOutMax=[]  NTsProdOutMin=[]  NTsProdOutMax=[]  UintegralTsProdOutMin=[]  UintegralTsProdOutMax=[]  UngainTsProdOutMin=[]  UngainTsProdOutMax=[]  ClampingZeroOutDataTypeStr=Inherit: Inherit via back propagation  ClampingZeroOutMin=[]  ClampingZeroOutMax=[]  FilterDenConstantOutDataTypeStr=Inherit: Inherit via back propagation  FilterDenConstantOutMin=[]  FilterDenConstantOutMax=[]  PCopyOutDataTypeStr=Inherit: Inherit via back propagation  PCopyOutMin=[]  PCopyOutMax=[]  NCopyOutDataTypeStr=Inherit: Inherit via back propagation  NCopyOutMin=[]  NCopyOutMax=[]  IntegratorContinuousStateAttributes=''  IntegratorStateMustResolveToSignalObject=off  IntegratorRTWStateStorageClass=Auto  FilterContinuousStateAttributes=''  FilterStateMustResolveToSignalObject=off  FilterRTWStateStorageClass=Auto  ParallelPVariant=InternalParameters  IdealPVariant=Disabled  IVariant=InternalParameters  DVariant=InternalParameters  IntegratorVariant=Continuous  SatVariant=Enabled  AWVariant=Passthrough  PCopyVariant=Disabled  TRVariant=Disabled  FdbkBlocksVariant=Forward  IdealPFdbkVariant=Disabled  SatFdbkVariant=Disabled  DerivativeFilterVariant=ContFilter  NVariant=InternalParameters  NCopyVariant=Disabled  FilterICVariant=InternalICsFilter  IntegratorICVariant=InternalICs  ExternalResetVariant=Disabled  TRSumVariant=Passthrough  SumFdbkVariant=Disabled  SumVariant=Sum_PID  TsampFilterVariant=InternalTs  TsampNgainVariant=Passthrough  TsampIntegralVariant=Disabled_SignalSpec  ExternalSaturationOutDataTypeStr=Inherit: Same as second input  DerivativeSourceVariant=ErrorSignal  PreIntVariant=InternalPreInt
  Postion Error [cm] : Scope
      settings: ActiveDisplayYMinimum=-12.877251579571915  ActiveDisplayYMaximum=12.868133706587805  DataLoggingVariableName=ScopeData15
  Pump 1 PWM PFI 14 (pin 1) : sldrtlib/Frequency Output  SampleTime=0.1  MaxMissedTicks=inf  ShowMissedTicks=off  YieldWhenWaiting=off  DrvName=National_Instruments/PCIe-6343  DrvAddress=4294967295  DrvOptions=[0 4479 48128 3 3 3 3]  Channels=3  FrequencySource=1  Frequency=100  FrequencyFinalValue=[]  DutySource=2  Duty=0  DutyFinalValue=0
      settings: AttributesFormatString=National Instruments\nPCIe-6343 [auto]
  Pump 1 direction P0.5 (pin 51) : sldrtlib/Digital Output  SampleTime=0.1  MaxMissedTicks=10  ShowMissedTicks=off  YieldWhenWaiting=off  DrvName=National_Instruments/PCIe-6343  DrvAddress=4294967295  DrvOptions=[0 4479 48128 3 3 3 3]  Channels=6  BitMode=1  InitialValue=1  FinalValue=1
      settings: AttributesFormatString=National Instruments\nPCIe-6343 [auto]
  Pump 2 PWM PFI 12 (pin 2) : sldrtlib/Frequency Output  SampleTime=0.1  MaxMissedTicks=inf  ShowMissedTicks=off  YieldWhenWaiting=off  DrvName=National_Instruments/PCIe-6343  DrvAddress=4294967295  DrvOptions=[0 4479 48128 3 3 3 3]  Channels=1  FrequencySource=1  Frequency=100  FrequencyFinalValue=[]  DutySource=2  Duty=0  DutyFinalValue=0
      settings: AttributesFormatString=National Instruments\nPCIe-6343 [auto]
  Pump 2 direction P0.1 (pin 17) : sldrtlib/Digital Output  SampleTime=0.1  MaxMissedTicks=10  ShowMissedTicks=off  YieldWhenWaiting=off  DrvName=National_Instruments/PCIe-6343  DrvAddress=4294967295  DrvOptions=[0 4479 48128 3 3 3 3]  Channels=2  BitMode=1  InitialValue=0  FinalValue=0
      settings: AttributesFormatString=National Instruments\nPCIe-6343 [auto]
  Pump displacement blend : MATLAB Function  TreatAsAtomicUnit=on
  Saturation : Saturate  UpperLimit=1  LowerLimit=0
  Saturation1 : Saturate  UpperLimit=1  LowerLimit=0
  Scope{,1..2,6} (4 alike) : Scope  NumInputPorts=2
      Scope settings: ActiveDisplayYMinimum=-1  ActiveDisplayYMaximum=1  DataLoggingSaveFormat=Array
      Scope1 settings: ActiveDisplayYMinimum=-0.093739718814631057  ActiveDisplayYMaximum=0.84365746933167962  DataLoggingVariableName=ScopeData10
      Scope2 settings: ActiveDisplayYMinimum=-1  ActiveDisplayYMaximum=1  DataLoggingVariableName=ScopeData11
      Scope6 settings: ActiveDisplayYMinimum=-0.14300210507249583  ActiveDisplayYMaximum=0.16495719400052031  DataLoggingVariableName=ScopeData21
  Scope4 : Scope
      settings: ActiveDisplayYMinimum=-0.30923958398617235  ActiveDisplayYMaximum=0.30923958398617235  DataLoggingVariableName=ScopeData16
  Sum : Sum  Inputs=|+-
  Sum1 : Sum  Inputs=|++
  Switch2 : Switch  Threshold=1  SaturateOnIntegerOverflow=off  InputSameDT=off
  Terminator : Terminator
  wires:
  Gain4/1 -> Commanded Flow [L/s]/1
  Gain3/1 -> Postion Error [cm]/1
  Gain2/1 -> Sum1/1, Scope/1
  Saturation1/1 -> Pump 1 direction P0.5 (pin 51)/1, Scope2/1
  Saturation/1 -> Pump 2 direction P0.1 (pin 17)/1, Scope2/2
  Demux/1 -> MATLAB Function/1(f)
  Demux/2 -> MATLAB Function2/1(f)
  Switch2/1 -> Demux/1
  Constant3/1 -> Switch2/3
  [WECmotionOnOff] -> Switch2/2
  Mux/1 -> Switch2/1
  Gain1/1 -> Sum1/2
  Flow rate limit for position control/1(Emulation piston flow rate) -> Divide1/1
  Sum1/1 -> Gain4/1, Flow rate limit for position control/1(flow rate cmd (m3/s))  "flow rate cmd (m3/s)"
  Pump displacement blend/2(f2) -> Mux/2
  Pump displacement blend/1(f1) -> Mux/1
  Constant4/1 -> MATLAB Function2/2(posCutIn)
  MATLAB Function2/2(dutySign) -> Saturation/1
  MATLAB Function2/1(dutyMag) -> Pump 2 PWM PFI 12 (pin 2)/1, Scope1/2
  Constant5/1 -> MATLAB Function2/3(negCutIn)
  Constant/1 -> MATLAB Function/2(posCutIn)
  Sum/1 -> PID Controller/1, Gain3/1
  Vel. meas. (m/s)/1 -> Terminator/1
  MATLAB Function/2(dutySign) -> Saturation1/1
  PID Controller/1 -> Gain2/1  "feedback cmd"
  Vel. ref. (m/s)/1 -> FF flowrate/1(vel)
  Pos. ref. (m)/1 -> Sum/1, Scope6/1
  Constant1/1 -> MATLAB Function/3(negCutIn)
  MATLAB Function/1(dutyMag) -> Pump 1 PWM PFI 14 (pin 1)/1, Scope1/1
  H1T shaft speed (rpm)/1 -> MATLAB Function1/1(speed_rpm)
  Divide1/1 -> Pump displacement blend/1(f), Scope4/1  "ave. frac. disp. cmd"
  Constant2/1 -> MATLAB Function1/2(numPumps)
  MATLAB Function1/1(maxFlow_m3perSec) -> Divide1/2
  Pos. meas. (m)/1 -> Sum/2, Scope6/2
  FF flowrate/1(flowrate) -> Scope/2, Gain1/1  "feedforward cmd"

== system SCADA/Charge Pump Control/Low-pressure manifold pressure control ==
  pressure ref. (Pa) : Inport
  pressure meas. (Pa) : Inport  Port=2
  PID Controller : slpidlib/PID Controller  Controller=PID  Form=Parallel  TimeDomain=Continuous-time  UseExternalTs=off  SampleTime=-1  IntegratorMethod=Forward Euler  FilterMethod=Forward Euler  ControllerParametersSource=internal  P=HIL_charge_kp  I=HIL_charge_ki  UseKiTs=off  D=0  UseExternalDerivativeSource=off  N=100  UseFilter=on  TunerSelectOption=Transfer Function Based (PID Tuner App)  InitialConditionSource=internal  InitialConditionForIntegrator=0  InitialConditionForFilter=0  DifferentiatorICPrevScaledInput=0  ExternalReset=none  TrackingMode=off  Kt=1  LimitOutput=off  SatLimitsSource=internal  UpperSaturationLimit=inf  LowerSaturationLimit=-inf  LinearizeAsGain=on  AntiWindupMode=none  Kb=1  LimitIntegrator=off  UpperIntegratorSaturationLimit=inf  LowerIntegratorSaturationLimit=-inf  POutMin=[]  POutMax=[]  IOutMin=[]  IOutMax=[]  DOutMin=[]  DOutMax=[]  NOutMin=[]  NOutMax=[]  SumOutMin=[]  SumOutMax=[]  SaturationOutMin=[]  SaturationOutMax=[]  PParamMin=[]  PParamMax=[]  IParamMin=[]  IParamMax=[]  DParamMin=[]  DParamMax=[]  NParamMin=[]  NParamMax=[]  KbParamMin=[]  KbParamMax=[]  KtParamMin=[]  KtParamMax=[]  KbOutMin=[]  KbOutMax=[]  KtOutMin=[]  KtOutMax=[]  IntegratorOutMin=[]  IntegratorOutMax=[]  FilterOutMin=[]  FilterOutMax=[]  SumI1OutMin=[]  SumI1OutMax=[]  SumI2OutMin=[]  SumI2OutMax=[]  SumI3OutMin=[]  SumI3OutMax=[]  SumI4OutMin=[]  SumI4OutMax=[]  SumDOutMin=[]  SumDOutMax=[]  DifferentiatorOutMin=[]  DifferentiatorOutMax=[]  FilterDiffOutCoefMin=[]  FilterDiffOutCoefMax=[]  ReciprocalOutMin=[]  ReciprocalOutMax=[]  SumDenOutMin=[]  SumDenOutMax=[]  SumNumOutMin=[]  SumNumOutMax=[]  DivideOutMin=[]  DivideOutMax=[]  UdiffTsProdOutMin=[]  UdiffTsProdOutMax=[]  NTsProdOutMin=[]  NTsProdOutMax=[]  UintegralTsProdOutMin=[]  UintegralTsProdOutMax=[]  UngainTsProdOutMin=[]  UngainTsProdOutMax=[]  ClampingZeroOutDataTypeStr=Inherit: Inherit via back propagation  ClampingZeroOutMin=[]  ClampingZeroOutMax=[]  FilterDenConstantOutDataTypeStr=Inherit: Inherit via back propagation  FilterDenConstantOutMin=[]  FilterDenConstantOutMax=[]  PCopyOutDataTypeStr=Inherit: Inherit via back propagation  PCopyOutMin=[]  PCopyOutMax=[]  NCopyOutDataTypeStr=Inherit: Inherit via back propagation  NCopyOutMin=[]  NCopyOutMax=[]  IntegratorContinuousStateAttributes=''  IntegratorStateMustResolveToSignalObject=off  IntegratorRTWStateStorageClass=Auto  FilterContinuousStateAttributes=''  FilterStateMustResolveToSignalObject=off  FilterRTWStateStorageClass=Auto  ParallelPVariant=InternalParameters  IdealPVariant=Disabled  IVariant=InternalParameters  DVariant=InternalParameters  IntegratorVariant=Continuous  SatVariant=Disabled  AWVariant=Passthrough  PCopyVariant=Disabled  TRVariant=Disabled  FdbkBlocksVariant=Forward  IdealPFdbkVariant=Disabled  SatFdbkVariant=Disabled  DerivativeFilterVariant=ContFilter  NVariant=InternalParameters  NCopyVariant=Disabled  FilterICVariant=InternalICsFilter  IntegratorICVariant=InternalICs  ExternalResetVariant=Disabled  TRSumVariant=Passthrough  SumFdbkVariant=Disabled  SumVariant=Sum_PID  TsampFilterVariant=InternalTs  TsampNgainVariant=Passthrough  TsampIntegralVariant=Disabled_SignalSpec  ExternalSaturationOutDataTypeStr=Inherit: Same as second input  DerivativeSourceVariant=ErrorSignal  PreIntVariant=InternalPreInt
  Speed Limits (FWD only) : Saturate  UpperLimit=HIL_charge_nMax  LowerLimit=HIL_charge_nMin
  Sum : Sum  Inputs=|+-
  charge pump shaft speed (rpm) : Outport
  wires:
  Sum/1 -> PID Controller/1
  PID Controller/1 -> Speed Limits (FWD only)/1  "feedback cmd"
  pressure ref. (Pa)/1 -> Sum/1
  pressure meas. (Pa)/1 -> Sum/2
  Speed Limits (FWD only)/1 -> charge pump shaft speed (rpm)/1

== system SCADA/Charge Pump Control/charge pump ==
  note: white
  Speed ref. : Inport
  Constant1 : Constant  Value=0
  FWD/REV P0.8 (pin 52) to VFD S2 : sldrtlib/Digital Output  SampleTime=0.1  MaxMissedTicks=10  ShowMissedTicks=off  YieldWhenWaiting=off  DrvName=National_Instruments/PCIe-6343  DrvAddress=4294967295  DrvOptions=[0 528767 48128 3 3 3 3]  Channels=9  BitMode=1  InitialValue=0  FinalValue=0
      settings: AttributesFormatString=National Instruments\nPCIe-6343 [auto]
  "Freq. reference AO 3 (pin 21) to VFD A1 " : sldrtlib/Analog Output  SampleTime=0.1  MaxMissedTicks=inf  ShowMissedTicks=off  YieldWhenWaiting=off  DrvName=National_Instruments/PCIe-6343  DrvAddress=4294967295  DrvOptions=[0 528767 48128 3 3 3 3]  Channels=4  RangeMode=1  VoltRange=1  InitialValue=0  FinalValue=0
      settings: AttributesFormatString=National Instruments\nPCIe-6343 [auto]
  Run/Stop P0.12 (pin 19) to VFD S1 : sldrtlib/Digital Output  SampleTime=0.1  MaxMissedTicks=10  ShowMissedTicks=off  YieldWhenWaiting=off  DrvName=National_Instruments/PCIe-6343  DrvAddress=4294967295  DrvOptions=[0 528767 48128 3 3 3 3]  Channels=13  BitMode=1  InitialValue=0  FinalValue=0
      settings: AttributesFormatString=National Instruments\nPCIe-6343 [auto]
  Scope{,1..3} (4 alike) : Scope
      Scope settings: ActiveDisplayYMinimum=-1  ActiveDisplayYMaximum=1  DataLoggingVariableName=ScopeData23
      Scope1 settings: ActiveDisplayYMinimum=6.3611111111111116  ActiveDisplayYMaximum=8.36111111111111  DataLoggingVariableName=ScopeData26
      Scope2 settings: ActiveDisplayYMinimum=6.3611111111111116  ActiveDisplayYMaximum=8.36111111111111  DataLoggingVariableName=ScopeData27
      Scope3 settings: ActiveDisplayYMinimum=6.3611111111111116  ActiveDisplayYMaximum=8.36111111111111  DataLoggingVariableName=ScopeData28
  freq. to voltage : Gain  Gain=10/HIL_charge_nMax*60
  rpm to freq. : Gain  Gain=1/60
  wires:
  Speed ref./1 -> Scope2/1, rpm to freq./1
  rpm to freq./1 -> Scope1/1, freq. to voltage/1
  [ChargePumpOnOff] -> Run/Stop P0.12 (pin 19) to VFD S1/1, Scope3/1
  freq. to voltage/1 -> Scope/1, "Freq. reference AO 3 (pin 21) to VFD A1 "/1
  Constant1/1 -> FWD/REV P0.8 (pin 52) to VFD S2/1

== system SCADA/ERU Control/ERU ==
  Speed ref. : Inport
  Constant : Constant  Value=0
  FWD/REV PFI 11/P2.3 (pin 46) to VFD S2 : sldrtlib/Digital Output  SampleTime=0.1  MaxMissedTicks=10  ShowMissedTicks=off  YieldWhenWaiting=off  DrvName=National_Instruments/PCIe-6343  DrvAddress=4294967295  DrvOptions=[0 528767 48128 3 3 3 3]  Channels=4  BitMode=1  InitialValue=[]  FinalValue=[]
      settings: AttributesFormatString=National Instruments\nPCIe-6343 [auto]
  "Freq. reference AO 0 (pin 22) to VFD A1 " : sldrtlib/Analog Output  SampleTime=0.1  MaxMissedTicks=inf  ShowMissedTicks=off  YieldWhenWaiting=off  DrvName=National_Instruments/PCIe-6343  DrvAddress=4294967295  DrvOptions=[0 528767 48128 3 3 3 3]  Channels=1  RangeMode=1  VoltRange=1  InitialValue=0  FinalValue=0
      settings: AttributesFormatString=National Instruments\nPCIe-6343 [auto]
  Run/Stop P0.3 (pin 47) to VFD S1 : sldrtlib/Digital Output  SampleTime=0.1  MaxMissedTicks=10  ShowMissedTicks=off  YieldWhenWaiting=off  DrvName=National_Instruments/PCIe-6343  DrvAddress=4294967295  DrvOptions=[0 528767 48128 3 3 3 3]  Channels=4  BitMode=1  InitialValue=[]  FinalValue=[]
      settings: AttributesFormatString=National Instruments\nPCIe-6343 [auto]
  Scope{,1..3} (4 alike) : Scope
      Scope settings: ActiveDisplayYMinimum=-1  ActiveDisplayYMaximum=1  DataLoggingVariableName=ScopeData8
      Scope1 settings: ActiveDisplayYMinimum=-1  ActiveDisplayYMaximum=1  DataLoggingVariableName=ScopeData9
      Scope2 settings: ActiveDisplayYMinimum=-1  ActiveDisplayYMaximum=1  DataLoggingVariableName=ScopeData7
      Scope3 settings: ActiveDisplayYMinimum=7.3333333333333339  ActiveDisplayYMaximum=9.3333333333333339  DataLoggingVariableName=ScopeData24
  freq. to voltage : Gain  Gain=10/HIL_ERU_nMax*60
  rpm to freq. : Gain  Gain=1/60
  wires:
  freq. to voltage/1 -> Scope/1, "Freq. reference AO 0 (pin 22) to VFD A1 "/1
  rpm to freq./1 -> Scope3/1, freq. to voltage/1
  Speed ref./1 -> Scope2/1, rpm to freq./1
  Constant/1 -> FWD/REV PFI 11/P2.3 (pin 46) to VFD S2/1
  [ERUOnOff] -> Scope1/1, Run/Stop P0.3 (pin 47) to VFD S1/1

== system SCADA/ERU Control/RO control ==
  recovery ref. : Inport
  recovery meas. : Inport  Port=2
  feed pressure (Pa) : Inport  Port=3
  PID Controller : slpidlib/PID Controller  Controller=PID  Form=Parallel  TimeDomain=Continuous-time  UseExternalTs=off  SampleTime=-1  IntegratorMethod=Forward Euler  FilterMethod=Forward Euler  ControllerParametersSource=internal  P=HIL_ERU_kp  I=HIL_ERU_ki  UseKiTs=off  D=HIL_ERU_kd  UseExternalDerivativeSource=off  N=100  UseFilter=on  TunerSelectOption=Transfer Function Based (PID Tuner App)  InitialConditionSource=internal  InitialConditionForIntegrator=0  InitialConditionForFilter=0  DifferentiatorICPrevScaledInput=0  ExternalReset=none  TrackingMode=off  Kt=1  LimitOutput=off  SatLimitsSource=internal  UpperSaturationLimit=inf  LowerSaturationLimit=-inf  LinearizeAsGain=on  AntiWindupMode=none  Kb=1  LimitIntegrator=off  UpperIntegratorSaturationLimit=inf  LowerIntegratorSaturationLimit=-inf  POutMin=[]  POutMax=[]  IOutMin=[]  IOutMax=[]  DOutMin=[]  DOutMax=[]  NOutMin=[]  NOutMax=[]  SumOutMin=[]  SumOutMax=[]  SaturationOutMin=[]  SaturationOutMax=[]  PParamMin=[]  PParamMax=[]  IParamMin=[]  IParamMax=[]  DParamMin=[]  DParamMax=[]  NParamMin=[]  NParamMax=[]  KbParamMin=[]  KbParamMax=[]  KtParamMin=[]  KtParamMax=[]  KbOutMin=[]  KbOutMax=[]  KtOutMin=[]  KtOutMax=[]  IntegratorOutMin=[]  IntegratorOutMax=[]  FilterOutMin=[]  FilterOutMax=[]  SumI1OutMin=[]  SumI1OutMax=[]  SumI2OutMin=[]  SumI2OutMax=[]  SumI3OutMin=[]  SumI3OutMax=[]  SumI4OutMin=[]  SumI4OutMax=[]  SumDOutMin=[]  SumDOutMax=[]  DifferentiatorOutMin=[]  DifferentiatorOutMax=[]  FilterDiffOutCoefMin=[]  FilterDiffOutCoefMax=[]  ReciprocalOutMin=[]  ReciprocalOutMax=[]  SumDenOutMin=[]  SumDenOutMax=[]  SumNumOutMin=[]  SumNumOutMax=[]  DivideOutMin=[]  DivideOutMax=[]  UdiffTsProdOutMin=[]  UdiffTsProdOutMax=[]  NTsProdOutMin=[]  NTsProdOutMax=[]  UintegralTsProdOutMin=[]  UintegralTsProdOutMax=[]  UngainTsProdOutMin=[]  UngainTsProdOutMax=[]  ClampingZeroOutDataTypeStr=Inherit: Inherit via back propagation  ClampingZeroOutMin=[]  ClampingZeroOutMax=[]  FilterDenConstantOutDataTypeStr=Inherit: Inherit via back propagation  FilterDenConstantOutMin=[]  FilterDenConstantOutMax=[]  PCopyOutDataTypeStr=Inherit: Inherit via back propagation  PCopyOutMin=[]  PCopyOutMax=[]  NCopyOutDataTypeStr=Inherit: Inherit via back propagation  NCopyOutMin=[]  NCopyOutMax=[]  IntegratorContinuousStateAttributes=''  IntegratorStateMustResolveToSignalObject=off  IntegratorRTWStateStorageClass=Auto  FilterContinuousStateAttributes=''  FilterStateMustResolveToSignalObject=off  FilterRTWStateStorageClass=Auto  ParallelPVariant=InternalParameters  IdealPVariant=Disabled  IVariant=InternalParameters  DVariant=InternalParameters  IntegratorVariant=Continuous  SatVariant=Disabled  AWVariant=Passthrough  PCopyVariant=Disabled  TRVariant=Disabled  FdbkBlocksVariant=Forward  IdealPFdbkVariant=Disabled  SatFdbkVariant=Disabled  DerivativeFilterVariant=ContFilter  NVariant=InternalParameters  NCopyVariant=Disabled  FilterICVariant=InternalICsFilter  IntegratorICVariant=InternalICs  ExternalResetVariant=Disabled  TRSumVariant=Passthrough  SumFdbkVariant=Disabled  SumVariant=Sum_PID  TsampFilterVariant=InternalTs  TsampNgainVariant=Passthrough  TsampIntegralVariant=Disabled_SignalSpec  ExternalSaturationOutDataTypeStr=Inherit: Same as second input  DerivativeSourceVariant=ErrorSignal  PreIntVariant=InternalPreInt
  Sum : Sum  Inputs=|+-
  Sum1 : Sum  Inputs=++|
  feed forward : MATLAB Function  TreatAsAtomicUnit=on
  ERU shaft speed (rpm) : Outport
  wires:
  Sum/1 -> PID Controller/1
  PID Controller/1 -> Sum1/2  "feedback cmd"
  recovery ref./1 -> feed forward/2(recoveryRef), Sum/1
  recovery meas./1 -> Sum/2
  feed pressure (Pa)/1 -> feed forward/1(pressure_feed)
  feed forward/1(shaftSpeedERU) -> Sum1/1
  Sum1/1 -> ERU shaft speed (rpm)/1

== system SCADA/Motor//Generator Control/RO feed pressure control ==
  feed pressure ref. (Pa) : Inport
  feed pressure meas. (Pa) : Inport  Port=2
  Feed forward : MATLAB Function  TreatAsAtomicUnit=on
  PID Controller : slpidlib/PID Controller  Controller=P  Form=Parallel  TimeDomain=Continuous-time  UseExternalTs=off  SampleTime=-1  IntegratorMethod=Forward Euler  FilterMethod=Forward Euler  ControllerParametersSource=internal  P=HIL_gen_kp  I=HIL_gen_ki  UseKiTs=off  D=HIL_gen_kd  UseExternalDerivativeSource=off  N=100  UseFilter=on  TunerSelectOption=Transfer Function Based (PID Tuner App)  InitialConditionSource=internal  InitialConditionForIntegrator=0  InitialConditionForFilter=0  DifferentiatorICPrevScaledInput=0  ExternalReset=none  TrackingMode=off  Kt=1  LimitOutput=off  SatLimitsSource=internal  UpperSaturationLimit=inf  LowerSaturationLimit=-inf  LinearizeAsGain=on  AntiWindupMode=none  Kb=1  LimitIntegrator=off  UpperIntegratorSaturationLimit=inf  LowerIntegratorSaturationLimit=-inf  POutMin=[]  POutMax=[]  IOutMin=[]  IOutMax=[]  DOutMin=[]  DOutMax=[]  NOutMin=[]  NOutMax=[]  SumOutMin=[]  SumOutMax=[]  SaturationOutMin=[]  SaturationOutMax=[]  PParamMin=[]  PParamMax=[]  IParamMin=[]  IParamMax=[]  DParamMin=[]  DParamMax=[]  NParamMin=[]  NParamMax=[]  KbParamMin=[]  KbParamMax=[]  KtParamMin=[]  KtParamMax=[]  KbOutMin=[]  KbOutMax=[]  KtOutMin=[]  KtOutMax=[]  IntegratorOutMin=[]  IntegratorOutMax=[]  FilterOutMin=[]  FilterOutMax=[]  SumI1OutMin=[]  SumI1OutMax=[]  SumI2OutMin=[]  SumI2OutMax=[]  SumI3OutMin=[]  SumI3OutMax=[]  SumI4OutMin=[]  SumI4OutMax=[]  SumDOutMin=[]  SumDOutMax=[]  DifferentiatorOutMin=[]  DifferentiatorOutMax=[]  FilterDiffOutCoefMin=[]  FilterDiffOutCoefMax=[]  ReciprocalOutMin=[]  ReciprocalOutMax=[]  SumDenOutMin=[]  SumDenOutMax=[]  SumNumOutMin=[]  SumNumOutMax=[]  DivideOutMin=[]  DivideOutMax=[]  UdiffTsProdOutMin=[]  UdiffTsProdOutMax=[]  NTsProdOutMin=[]  NTsProdOutMax=[]  UintegralTsProdOutMin=[]  UintegralTsProdOutMax=[]  UngainTsProdOutMin=[]  UngainTsProdOutMax=[]  ClampingZeroOutDataTypeStr=Inherit: Inherit via back propagation  ClampingZeroOutMin=[]  ClampingZeroOutMax=[]  FilterDenConstantOutDataTypeStr=Inherit: Inherit via back propagation  FilterDenConstantOutMin=[]  FilterDenConstantOutMax=[]  PCopyOutDataTypeStr=Inherit: Inherit via back propagation  PCopyOutMin=[]  PCopyOutMax=[]  NCopyOutDataTypeStr=Inherit: Inherit via back propagation  NCopyOutMin=[]  NCopyOutMax=[]  IntegratorContinuousStateAttributes=''  IntegratorStateMustResolveToSignalObject=off  IntegratorRTWStateStorageClass=Auto  FilterContinuousStateAttributes=''  FilterStateMustResolveToSignalObject=off  FilterRTWStateStorageClass=Auto  ParallelPVariant=InternalParameters  IdealPVariant=Disabled  IVariant=Disabled  DVariant=Disabled  IntegratorVariant=Disabled  SatVariant=Disabled  AWVariant=Disabled  PCopyVariant=Disabled  TRVariant=Disabled  FdbkBlocksVariant=Forward  IdealPFdbkVariant=Disabled  SatFdbkVariant=Disabled  DerivativeFilterVariant=Disabled  NVariant=Disabled  NCopyVariant=Disabled_SignalSpec  FilterICVariant=Disabled  IntegratorICVariant=Disabled  ExternalResetVariant=Disabled  TRSumVariant=Passthrough  SumFdbkVariant=Disabled  SumVariant=Passthrough_P  TsampFilterVariant=InternalTs  TsampNgainVariant=Passthrough  TsampIntegralVariant=Disabled_SignalSpec  ExternalSaturationOutDataTypeStr=Inherit: Same as second input  DerivativeSourceVariant=Disabled  PreIntVariant=InternalPreInt
  Speed Limits (FWD only) : Saturate  UpperLimit=HIL_gen_nMax  LowerLimit=HIL_gen_nMin
  Sum : Sum  Inputs=|+-
  Sum1 : Sum  Inputs=++|
  gen shaft speed (rpm) : Outport
  wires:
  Sum/1 -> ?
  ? -> Sum1/2  "feedback cmd"
  feed pressure ref. (Pa)/1 -> Feed forward/1(p), Sum/1
  feed pressure meas. (Pa)/1 -> Sum/2
  Speed Limits (FWD only)/1 -> gen shaft speed (rpm)/1
  Sum1/1 -> Speed Limits (FWD only)/1
  Feed forward/1(shaftSpeed_ff) -> Sum1/1

== system SCADA/Motor//Generator Control/generator ==
  Speed ref. : Inport
  run/stop : Inport  Port=2
  fwd/rev : Inport  Port=3
  FWD/REV P0.0 (pin 52) to VFD S2 : sldrtlib/Digital Output  SampleTime=0.1  MaxMissedTicks=10  ShowMissedTicks=off  YieldWhenWaiting=off  DrvAddress=0  DrvOptions=0  Channels=1  BitMode=1  InitialValue=[]  FinalValue=[]
  "Freq. reference AO 1 (pin 21) to VFD A1 " : daqlib/Analog Output  DeviceMenu=ni Dev1 (PCIe-6343)  Device=(none)  ObjConstructor=daq.createSession('ni')  NChannelsSelected=1  Channels=1$ao0$$Dev1$1$1$N/A$#1$ao1$$Dev1$1$1$N/A$#1$ao2$$Dev1$1$1$N/A$#1$ao3$$Dev1$1$1$N/A$#  NPorts=1 for all channels  SampleRate=0  ActualRate=0
  Run/Stop P0.4 (pin 19) to VFD S1 : sldrtlib/Digital Output  SampleTime=0.1  MaxMissedTicks=10  ShowMissedTicks=off  YieldWhenWaiting=off  DrvAddress=0  DrvOptions=0  Channels=1  BitMode=1  InitialValue=[]  FinalValue=[]
  freq. to voltage1 : Gain  Gain=10/HIL_gen_nMax
  rpm to freq.1 : Gain  Gain=1/60
  wires:
  Speed ref./1 -> rpm to freq.1/1
  run/stop/1 -> ?
  fwd/rev/1 -> ?
  rpm to freq.1/1 -> freq. to voltage1/1
  freq. to voltage1/1 -> "Freq. reference AO 1 (pin 21) to VFD A1 "/1

== system SCADA/Prescribed Motion/Constant Position ==
  Constant : Constant  Value=0
  pos. ref. : Outport
  vel. ref. : Outport  Port=2
  wires:
  [NomPosition_WECpump] -> pos. ref./1
  Constant/1 -> vel. ref./1

== system SCADA/Prescribed Motion/Constant WEC-driven Pump Flow1 ==
  Gain : Gain  Gain=-1/HIL_WECpump_A_rod
  Gain1 : Gain  Gain=1/HIL_WECpump_A_cap
  Integrator : Integrator
  State Transition Table : State Transition Table  TreatAsAtomicUnit=on
  Switch : Switch  Criteria=u2 > Threshold  SaturateOnIntegerOverflow=off  InputSameDT=off
  pos. ref. : Outport
  vel. ref. : Outport  Port=2
  wires:
  Gain1/1 -> Switch/1
  Switch/1 -> vel. ref./1, Integrator/1
  Gain/1 -> Switch/3
  [NomFlow_WECpump] -> Gain1/1, Gain/1
  Integrator/1 -> State Transition Table/1(pos), pos. ref./1
  State Transition Table/1(direction) -> Switch/2

== system SCADA/Prescribed Motion/Prescribed Wave-like Motion ==
  Clock : Clock
  Derivative : Derivative
  Gain : Gain  Gain=2*pi
  Math Function : Math  Operator=reciprocal
  Wave-like motion : MATLAB Function  TreatAsAtomicUnit=on
  pos. ref. : Outport
  vel. ref. : Outport  Port=2
  wires:
  [NomFlow_WECpump] -> Wave-like motion/2(meanFlow)
  Wave-like motion/1(pos) -> Derivative/1, pos. ref./1
  Derivative/1 -> vel. ref./1
  Clock/1 -> Wave-like motion/1(t)
  [T_p] -> Math Function/1
  Math Function/1 -> Gain/1
  Gain/1 -> Wave-like motion/3(w)
  [WECmotionType] -> Wave-like motion/4(WECmotionType)
